simulink model "pendcarthil"  (Simulink 8.9)
settings: Solver=FixedStepAuto  StartTime=0.0  StopTime=tsim  RelTol=1e-3  EnableMultiTasking=on
values from neighbouring files (symbols this model uses):
  T = 0.01    [discretise_cascade.m]    (also in pendcarthilsim.m)
  theta0 = 5*pi/180    (= 0.0872664625997)    [pendcarthilsim.m]
undefined symbols (not defined in the file or in its folder): param
libraries: instrumentlib x4
settings Model: Creator=Chris  LastModifiedBy=Patrick
settings SolverCC: AlgebraicLoopSolver=LineSearch
settings OptimizationCC: ExpressionDepthLimit=2147483647  InitFltsAndDblsToZero=on
settings DebuggingCC: AlgebraicLoopMsg=none  SaveWithParameterizedLinksMsg=none
settings GRTTargetCC: TargetFcnLib=ansi_tfl_tmw.mat

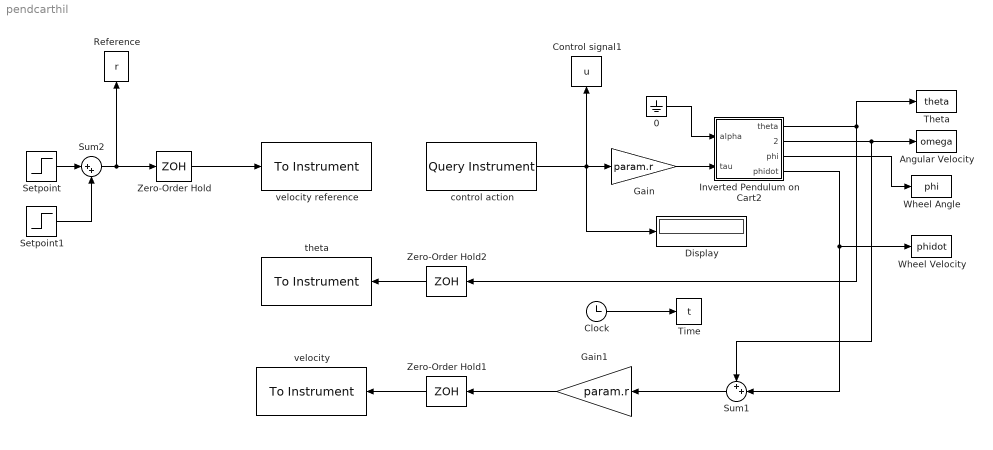
== system pendcarthil ==
  0 : Ground
  Angular Velocity : ToWorkspace  VariableName=omega  SampleTime=-1
  Clock : Clock
  Control signal1 : ToWorkspace  VariableName=u  SampleTime=-1
  Display : Display
  Gain : Gain  Gain=param.r  OutMax=1
  Gain1 : Gain  Gain=param.r  OutMax=1
  Inverted Pendulum on Cart2 : Subsystem
  Reference : ToWorkspace  VariableName=r  SampleTime=-1
  Setpoint : Step  Time=10  After=0.5  SampleTime=0
  Setpoint1 : Step  Time=20  After=-0.5  SampleTime=0
  Sum1 : Sum  Inputs=++|
  Sum2 : Sum  Inputs=|++
  Theta : ToWorkspace  VariableName=theta  SampleTime=-1
  Time : ToWorkspace  VariableName=t  SampleTime=-1
  Wheel Angle : ToWorkspace  VariableName=phi  SampleTime=-1
  Wheel Velocity : ToWorkspace  VariableName=phidot  SampleTime=-1
  Zero-Order Hold : ZeroOrderHold  SampleTime=T
  Zero-Order Hold1 : ZeroOrderHold  SampleTime=T
  Zero-Order Hold2 : ZeroOrderHold  SampleTime=T
  control action : instrumentlib/Query Instrument  sampleTime=T  isWorkspaceObject=off  timeout=10  inputBufferSize=512  protocol=Serial  serialPort=COM4  baudRate=115200  gpibVendor=Agilent Technologies  boardIndex=0  primaryAddress=1  secondaryAddress=0  visaVendor=Agilent  visaSerialPort=0  chassisIndex=0  logicalAddress=0  tcpRemoteHost='127.0.0.1'  tcpRemotePort=4500  udpRemoteHost='127.0.0.1'  udpRemotePort=9090  visaTCPBoardIndex=0  visaTCPRemoteHost='127.0.0.1'  usbBoardIndex=0  usbManufID=0  usbModelCode=0  usbSerialNumber=0  initAction=None  initCommand='DATA:SOURCE CH1'  initFunction=get  queryCommand='ctrl\n'  responseFormat=ASCII  asciiFormatting='%g\n'  precision=8-bit integer  byteOrder=Little endian  valuesToRead=1  removeBytes=off  afterOutputAction=Repeat query for new data  enableFrames=off  frameSize=1
      settings: SourceProductName=Instrument Control Toolbox  SourceProductBaseCode=IC
  theta : instrumentlib/To Instrument  sampleTime=T  isWorkspaceObject=off  timeout=10  inputBufferSize=8192  protocol=Serial  serialPort=COM4  baudRate=115200  gpibVendor=Agilent Technologies  boardIndex=0  primaryAddress=1  secondaryAddress=0  visaVendor=Agilent  visaSerialPort=0  chassisIndex=0  logicalAddress=0  tcpRemoteHost='127.0.0.1'  tcpRemotePort=4500  udpRemoteHost='127.0.0.1'  udpRemotePort=9090  visaTCPBoardIndex=0  visaTCPRemoteHost='127.0.0.1'  usbBoardIndex=0  usbManufID=0  usbModelCode=0  usbSerialNumber=0  initAction=None  initCommand='DATA:SOURCE CH1'  initFunction=get  command=''  sendFormat=ASCII  asciiFormatting='set theta %g\n'  precision=8-bit integer  byteOrder=Little endian
      settings: SourceProductName=Instrument Control Toolbox  SourceProductBaseCode=IC
  velocity : instrumentlib/To Instrument  sampleTime=T  isWorkspaceObject=off  timeout=10  inputBufferSize=8192  protocol=Serial  serialPort=COM4  baudRate=115200  gpibVendor=Agilent Technologies  boardIndex=0  primaryAddress=1  secondaryAddress=0  visaVendor=Agilent  visaSerialPort=0  chassisIndex=0  logicalAddress=0  tcpRemoteHost='127.0.0.1'  tcpRemotePort=4500  udpRemoteHost='127.0.0.1'  udpRemotePort=9090  visaTCPBoardIndex=0  visaTCPRemoteHost='127.0.0.1'  usbBoardIndex=0  usbManufID=0  usbModelCode=0  usbSerialNumber=0  initAction=None  initCommand='DATA:SOURCE CH1'  initFunction=get  command=''  sendFormat=ASCII  asciiFormatting='set v %g\n'  precision=8-bit integer  byteOrder=Little endian
      settings: SourceProductName=Instrument Control Toolbox  SourceProductBaseCode=IC
  velocity reference : instrumentlib/To Instrument  sampleTime=-1  isWorkspaceObject=off  timeout=10  inputBufferSize=8192  protocol=Serial  serialPort=COM4  baudRate=115200  gpibVendor=Agilent Technologies  boardIndex=0  primaryAddress=1  secondaryAddress=0  visaVendor=Agilent  visaSerialPort=0  chassisIndex=0  logicalAddress=0  tcpRemoteHost='127.0.0.1'  tcpRemotePort=4500  udpRemoteHost='127.0.0.1'  udpRemotePort=9090  visaTCPBoardIndex=0  visaTCPRemoteHost='127.0.0.1'  usbBoardIndex=0  usbManufID=0  usbModelCode=0  usbSerialNumber=0  initAction=None  initCommand='DATA:SOURCE CH1'  initFunction=get  command=''  sendFormat=ASCII  asciiFormatting='set vref %g\n'  precision=8-bit integer  byteOrder=Little endian
      settings: SourceProductName=Instrument Control Toolbox  SourceProductBaseCode=IC
  wires:
  Clock/1 -> Time/1
  Inverted Pendulum on Cart2/1(theta) -> Zero-Order Hold2/1, Theta/1
  Inverted Pendulum on Cart2/2(omega) -> Sum1/1, Angular Velocity/1
  Setpoint/1 -> Sum2/1
  Setpoint1/1 -> Sum2/2
  Sum2/1 -> Zero-Order Hold/1, Reference/1
  0/1 -> Inverted Pendulum on Cart2/1(alpha)
  control action/1 -> Display/1, Gain/1, Control signal1/1
  Gain/1 -> Inverted Pendulum on Cart2/2(tau)
  Inverted Pendulum on Cart2/3(phi) -> Wheel Angle/1
  Inverted Pendulum on Cart2/4(phidot) -> Wheel Velocity/1, Sum1/2
  Sum1/1 -> Gain1/1
  Gain1/1 -> Zero-Order Hold1/1
  Zero-Order Hold1/1 -> velocity/1
  Zero-Order Hold2/1 -> theta/1
  Zero-Order Hold/1 -> velocity reference/1

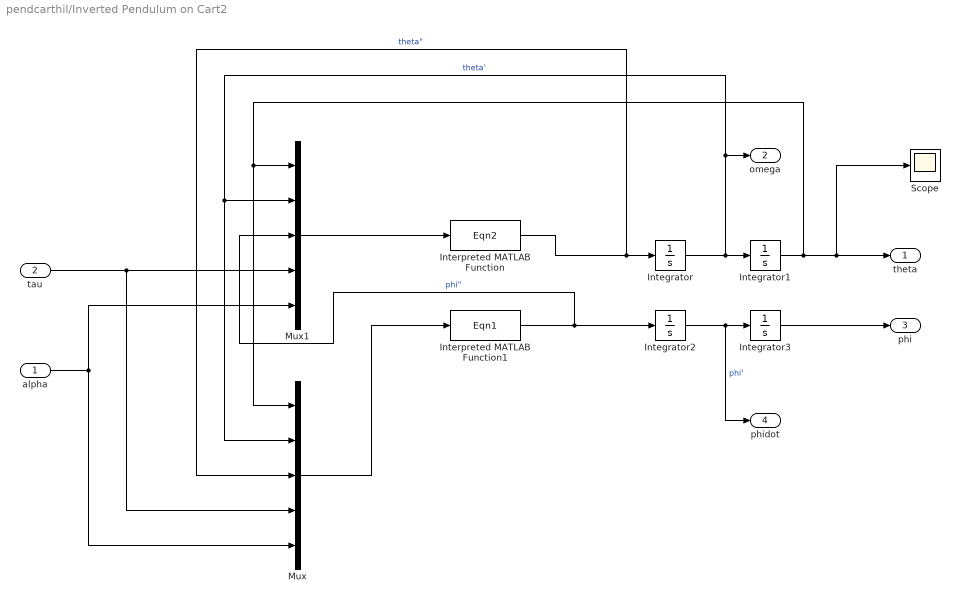
== system pendcarthil/Inverted Pendulum on Cart2 ==
  alpha : Inport
  tau : Inport  Port=2
  Integrator : Integrator
  Integrator1 : Integrator  InitialCondition=theta0
  Integrator2 : Integrator
  Integrator3 : Integrator
  Interpreted MATLAB Function : MATLABFcn  MATLABFcn=Eqn2  OutputDimensions=1  Output1D=off
  Interpreted MATLAB Function1 : MATLABFcn  MATLABFcn=Eqn1  OutputDimensions=1  Output1D=off
  Mux : Mux  Inputs=[1 1 1 1 1]
  Mux1 : Mux  Inputs=[1 1 1 1 1]
  Scope : Scope
  theta : Outport
  omega : Outport  Port=2
  phi : Outport  Port=3
  phidot : Outport  Port=4
  wires:
  Integrator/1 -> Integrator1/1, Mux1/2, Mux/2, omega/1  "theta'"
  Integrator2/1 -> Integrator3/1, phidot/1  "phi'"
  alpha/1 -> Mux1/5, Mux/5
  Integrator3/1 -> phi/1
  Interpreted MATLAB Function/1 -> Mux/3, Integrator/1  "theta\""
  Interpreted MATLAB Function1/1 -> Mux1/3, Integrator2/1  "phi\""
  tau/1 -> Mux/4, Mux1/4
  Mux1/1 -> Interpreted MATLAB Function/1
  Integrator1/1 -> Mux1/1, Mux/1, Scope/1, theta/1
  Mux/1 -> Interpreted MATLAB Function1/1
